simulink library "relay_ANSI_F25_lib"  (Simulink 8.1)
settings: Solver=ode45  StartTime=0.0  StopTime=10.0  RelTol=1e-3
undefined symbols (not defined in the file or in its folder): angle_threshold, dF_threshold, dV_threshold, Ts, VRMSLL
libraries: powerlib_extras x6, simulink_extras x5, simulink x5, dspsigops x2, RMS_lib x1
settings Model: Creator=RE25624  LastModifiedBy=hptb1

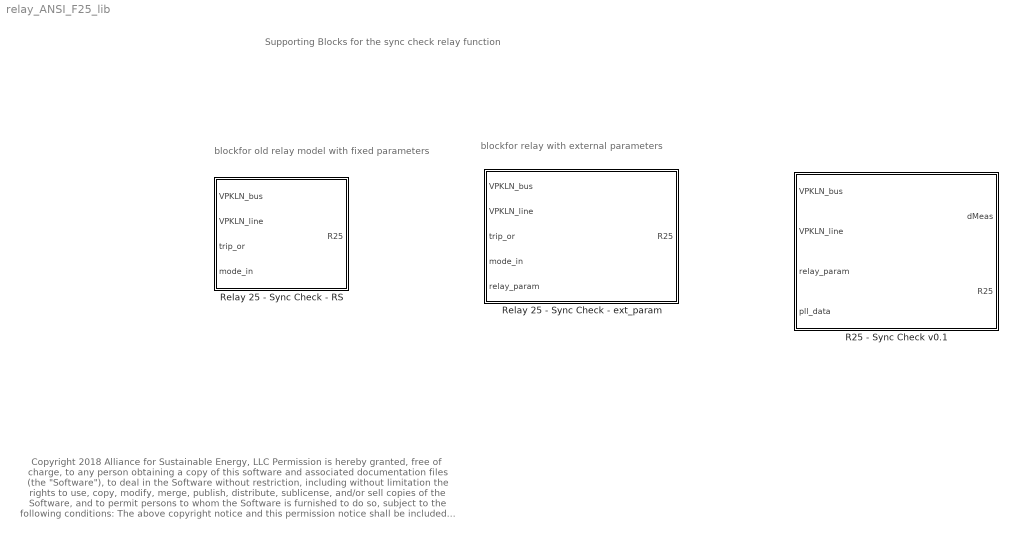
== system relay_ANSI_F25_lib ==
  note: blockfor relay with external parameters
  note: Supporting Blocks for the sync check relay function
  note: blockfor old relay model with fixed parameters
  note: Copyright 2018 Alliance for Sustainable Energy, LLC
      |
      | Permission is hereby granted, free of charge, to any person obtaining a copy of this software
      | and associated documentation files (the "Software"), to deal in the Software without restriction,
      | including without limitation the rights to use, copy, modify, merge, publish, distribute, sublicense,
      | and/or sell copies of the Software, and to permit persons to whom the Software is furnished to do so,
      | subject to the following conditions:
      |
      | The above copyright notice and this permission notice shall be included in all copies or substantial portions of the Software.
      |
      | THE SOFTWARE IS PROVIDED "AS IS", WITHOUT WARRANTY OF ANY KIND, EXPRESS OR IMPLIED, INCLUDING
      | BUT NOT LIMITED TO THE WARRANTIES OF MERCHANTABILITY, FITNESS FOR A PARTICULAR PURPOSE AND
      | NONINFRINGEMENT. IN NO EVENT SHALL THE AUTHORS, THE COPYRIGHT HOLDERS, THE UNITED STATES,
      | THE UNITED STATES DEPARTMENT OF ENERGY, OR ANY OF THEIR EMPLOYEES BE LIABLE FOR ANY CLAIM,
      | DAMAGES OR OTHER LIABILITY, WHETHER IN AN ACTION OF CONTRACT, TORT OR OTHERWISE, ARISING FROM,
      | OUT OF OR IN CONNECTION WITH THE SOFTWARE OR THE USE OR OTHER DEALINGS IN THE SOFTWARE.
  R25 - Sync Check v0.1 : Subsystem  mask(Relay synch check){Ts=Ts}
      mask prompts: Ts "Sampling Time [Sec]"
      mask help:
      | This block checks if the the specified conditions for breaker reclosing
      | are met at both terminals of the circuit breaker. This synch check is
      | intended for use in bus-ties, and service lines.
      |
      | The input bus with the relay parameters should be ordered as follows:
      | 1) VRMSLL
      | 2) IOC
      | 3) TOC
      | 4) dV_threshold
      | 5) angle_threshold
      | 6) dF_threshold
  Relay 25 - Sync Check - RS : Subsystem  mask{VRMSLL=VRMSLL, Ts=Ts, dV_threshold=dV_threshold, angle_threshold=angle_threshold, dF_threshold=dF_threshold}
      mask prompts: VRMSLL "Nominal Voltage [VRMSLL]"; Ts "Sampling Time [Sec]"; dV_threshold "Percent Voltage Threshold [%]"; angle_threshold "Angle Threshold [degress]"; dF_threshold "Frequency Threshold [Hz]"
  Relay 25 - Sync Check - ext_param : Subsystem  mask(Relay synch check){Ts=Ts}
      mask prompts: Ts "Sampling Time [Sec]"
      mask help:
      | This block checks if the the specified conditions for breaker reclosing
      | are met at both terminals of the circuit breaker. This synch check is
      | intended for use in bus-ties, and service lines.
      |
      | The input bus with the relay parameters should be ordered as follows:
      | 1) VRMSLL
      | 2) IOC
      | 3) TOC
      | 4) dV_threshold
      | 5) angle_threshold
      | 6) dF_threshold

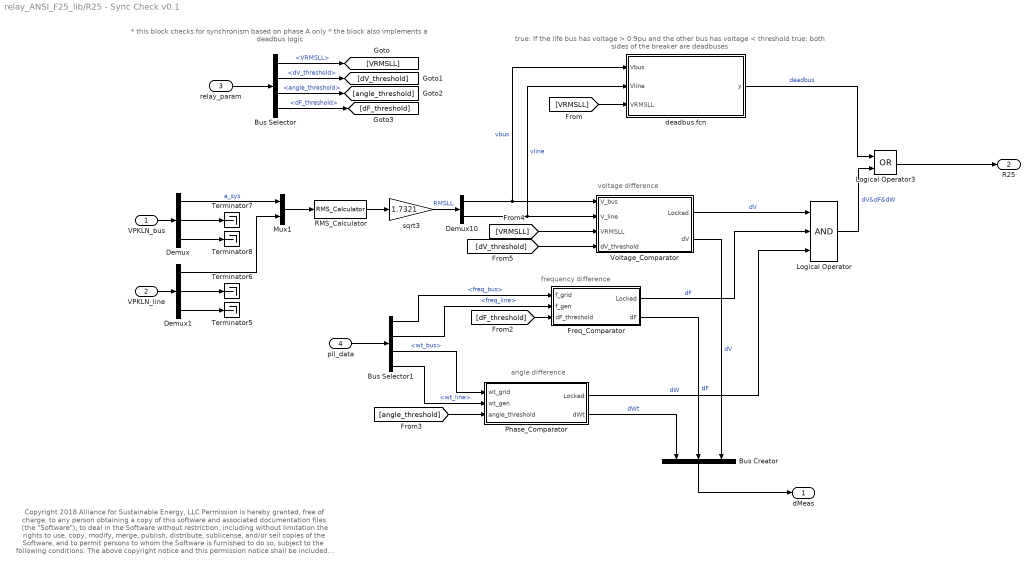
== system relay_ANSI_F25_lib/R25 - Sync Check v0.1 ==
  note: Copyright 2018 Alliance for Sustainable Energy, LLC
      |
      | Permission is hereby granted, free of charge, to any person obtaining a copy of this software
      | and associated documentation files (the "Software"), to deal in the Software without restriction,
      | including without limitation the rights to use, copy, modify, merge, publish, distribute, sublicense,
      | and/or sell copies of the Software, and to permit persons to whom the Software is furnished to do so,
      | subject to the following conditions:
      |
      | The above copyright notice and this permission notice shall be included in all copies or substantial portions of the Software.
      |
      | THE SOFTWARE IS PROVIDED "AS IS", WITHOUT WARRANTY OF ANY KIND, EXPRESS OR IMPLIED, INCLUDING
      | BUT NOT LIMITED TO THE WARRANTIES OF MERCHANTABILITY, FITNESS FOR A PARTICULAR PURPOSE AND
      | NONINFRINGEMENT. IN NO EVENT SHALL THE AUTHORS, THE COPYRIGHT HOLDERS, THE UNITED STATES,
      | THE UNITED STATES DEPARTMENT OF ENERGY, OR ANY OF THEIR EMPLOYEES BE LIABLE FOR ANY CLAIM,
      | DAMAGES OR OTHER LIABILITY, WHETHER IN AN ACTION OF CONTRACT, TORT OR OTHERWISE, ARISING FROM,
      | OUT OF OR IN CONNECTION WITH THE SOFTWARE OR THE USE OR OTHER DEALINGS IN THE SOFTWARE.
  note: true: If the life bus has voltage > 0.9pu and the other bus has voltage < threshold
      | true: both sides of the breaker are deadbuses
  note: voltage difference
  note: frequency difference
  note: angle difference
  note: * this block checks for synchronism based on phase A only
      | * the block also implements a deadbus logic
  VPKLN_bus : Inport
  VPKLN_line : Inport  Port=2
  relay_param : Inport  Port=3
  pll_data : Inport  Port=4
  Bus Creator : BusCreator  Inputs=3
  Bus Selector : BusSelector  OutputSignals=VRMSLL,dV_threshold,angle_threshold,dF_threshold
  Bus Selector1 : BusSelector  OutputSignals=freq_bus,freq_line,wt_bus,wt_line
  Demux : Demux  Outputs=3
  Demux1 : Demux  Outputs=3
  Demux10 : Demux  Outputs=2
  Freq_Comparator : Subsystem
  Logical Operator : Logic  Inputs=3  AllPortsSameDT=off  OutDataTypeStr=boolean
  Logical Operator3 : Logic  Operator=OR  AllPortsSameDT=off  OutDataTypeStr=boolean
  Mux1 : Mux  Inputs=2
  Phase_Comparator : Subsystem
  RMS_Calculator : RMS_lib/RMS_Calculator  Ts=Ts
  Terminator{5..8} (4 alike) : Terminator
  Voltage_Comparator : Subsystem
  deadbus fcn : MATLAB Function  TreatAsAtomicUnit=on
  sqrt3 : Gain  Gain=1.7321
  dMeas : Outport
  R25 : Outport  Port=2
  wires:
  Logical Operator3/1 -> R25/1
  pll_data/1 -> Bus Selector1/1
  Logical Operator/1 -> Logical Operator3/2  "dV&dF&dW"
  deadbus fcn/1(y) -> Logical Operator3/1  "deadbus"
  VPKLN_line/1 -> Demux1/1
  VPKLN_bus/1 -> Demux/1
  Demux/3 -> Terminator8/1
  Demux/2 -> Terminator7/1
  Demux1/3 -> Terminator5/1
  Demux1/2 -> Terminator6/1
  Demux1/1 -> Mux1/2
  Demux/1 -> Mux1/1  "a_sys"
  Demux10/1 -> Voltage_Comparator/1(V_bus), deadbus fcn/1(Vbus)  "vbus"
  Bus Selector1/1 -> Freq_Comparator/1(f_grid)  "<freq_bus>"
  Bus Selector1/2 -> Freq_Comparator/2(f_gen)  "<freq_line>"
  Bus Selector1/3 -> Phase_Comparator/1(wt_grid)  "<wt_bus>"
  Bus Selector1/4 -> Phase_Comparator/2(wt_gen)  "<wt_line>"
  Demux10/2 -> Voltage_Comparator/2(V_line), deadbus fcn/2(Vline)  "vline"
  Voltage_Comparator/1(Locked) -> Logical Operator/1  "dV"
  Freq_Comparator/1(Locked) -> Logical Operator/2  "dF"
  Phase_Comparator/1(Locked) -> Logical Operator/3  "dW"
  RMS_Calculator/1 -> sqrt3/1
  Mux1/1 -> RMS_Calculator/1
  sqrt3/1 -> Demux10/1  "RMSLL"
  [VRMSLL] -> deadbus fcn/3(VRMSLL)
  relay_param/1 -> Bus Selector/1
  Bus Selector/1 -> [VRMSLL]  "<VRMSLL>"
  Bus Selector/2 -> [dV_threshold]  "<dV_threshold>"
  Bus Selector/3 -> [angle_threshold]  "<angle_threshold>"
  Bus Selector/4 -> [dF_threshold]  "<dF_threshold>"
  [dF_threshold] -> Freq_Comparator/3(dF_threshold)
  [angle_threshold] -> Phase_Comparator/3(angle_threshold)
  [VRMSLL] -> Voltage_Comparator/3(VRMSLL)
  [dV_threshold] -> Voltage_Comparator/4(dV_threshold)
  Voltage_Comparator/2(dV) -> Bus Creator/3  "dV"
  Freq_Comparator/2(dF) -> Bus Creator/2  "dF"
  Phase_Comparator/2(dWt) -> Bus Creator/1  "dWt"
  Bus Creator/1 -> dMeas/1

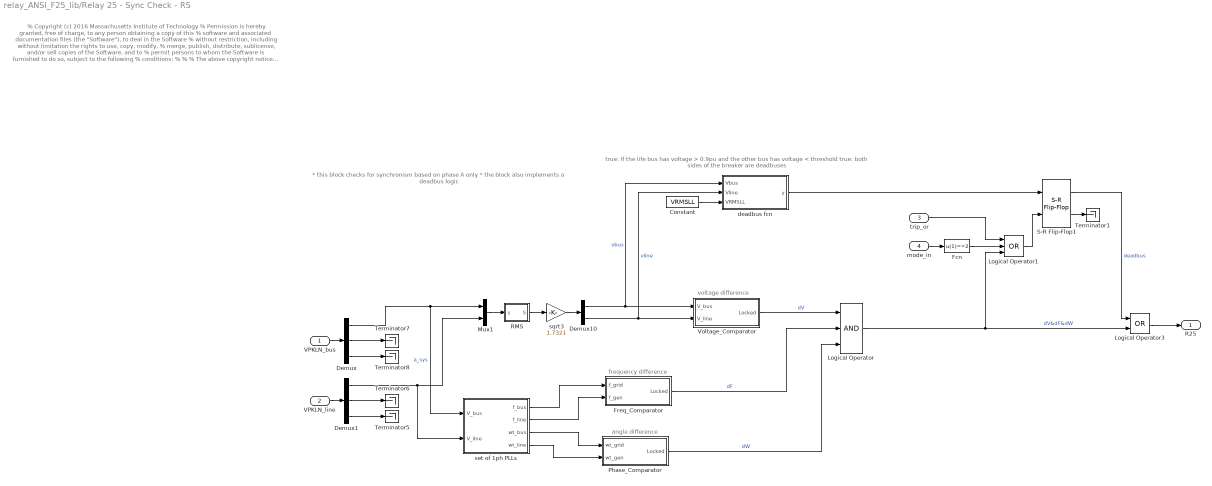
== system relay_ANSI_F25_lib/Relay 25 - Sync Check - RS ==
  note: * this block checks for synchronism based on phase A only
      | * the block also implements a deadbus logic
  note: angle difference
  note: frequency difference
  note: voltage difference
  note: true: If the life bus has voltage > 0.9pu and the other bus has voltage < threshold
      | true: both sides of the breaker are deadbuses
  note: % Copyright (c) 2016 Massachusetts Institute of Technology
      | % Permission is hereby granted, free of charge, to any person obtaining a copy of this
      | % software and associated documentation files (the "Software"), to deal in the Software
      | % without restriction, including without limitation the rights to use, copy, modify,
      | % merge, publish, distribute, sublicense, and/or sell copies of the Software, and to
      | % permit persons to whom the Software is furnished to do so, subject to the following
      | % conditions:
      | %
      | %
      | % The above copyright notice and this permission notice shall be included in
      | % all copies or substantial portions of the Software.
      | %
      | % THE SOFTWARE IS PROVIDED "AS IS", WITHOUT WARRANTY OF ANY KIND, EXPRESS OR IMPLIED,
      | % INCLUDING BUT NOT LIMITED TO THE WARRANTIES OF MERCHANTABILITY, FITNESS FOR A
      | % PARTICULAR PURPOSE AND NONINFRINGEMENT. IN NO EVENT SHALL THE AUTHORS OR COPYRIGHT
      | % HOLDERS BE LIABLE FOR ANY CLAIM, DAMAGES OR OTHER LIABILITY, WHETHER IN AN ACTION
      | % OF CONTRACT, TORT OR OTHERWISE, ARISING FROM, OUT OF OR IN CONNECTION WITH THE
      | % SOFTWARE OR THE USE OR OTHER DEALINGS IN THE SOFTWARE.
      | %
      | %
      | %%
  VPKLN_bus : Inport
  VPKLN_line : Inport  Port=2
  trip_or : Inport  Port=3
  mode_in : Inport  Port=4
  Constant : Constant  Value=VRMSLL
  Demux : Demux  Outputs=3
  Demux1 : Demux  Outputs=3
  Demux10 : Demux  Outputs=2
  Fcn : Fcn  Expr=u(1)==2
  Freq_Comparator : Subsystem
  Logical Operator : Logic  Inputs=3  AllPortsSameDT=off  OutDataTypeStr=boolean
  Logical Operator1 : Logic  Operator=OR  Inputs=3  AllPortsSameDT=off  OutDataTypeStr=boolean
  Logical Operator3 : Logic  Operator=OR  AllPortsSameDT=off  OutDataTypeStr=boolean
  Mux1 : Mux  Inputs=2
  Phase_Comparator : Subsystem
  RMS : Subsystem
  S-R Flip-Flop1 : simulink_extras/Flip Flops/S-R Flip-Flop  initial_condition=0
  Terminator{1,5..8} (5 alike) : Terminator
  Voltage_Comparator : Subsystem
  deadbus fcn : MATLAB Function  TreatAsAtomicUnit=on
  set of 1ph PLLs : Subsystem
  sqrt3 : Gain  Gain=1.7321
  R25 : Outport
  wires:
  Fcn/1 -> Logical Operator1/2
  mode_in/1 -> Fcn/1
  trip_or/1 -> Logical Operator1/1
  Logical Operator1/1 -> S-R Flip-Flop1/2
  deadbus fcn/1(y) -> S-R Flip-Flop1/1
  S-R Flip-Flop1/1 -> Logical Operator3/1  "deadbus"
  Logical Operator3/1 -> R25/1
  S-R Flip-Flop1/2 -> Terminator1/1
  Constant/1 -> deadbus fcn/3(VRMSLL)
  sqrt3/1 -> Demux10/1
  Mux1/1 -> RMS/1(s)
  RMS/1(S) -> sqrt3/1
  Phase_Comparator/1(Locked) -> Logical Operator/3  "dW"
  Freq_Comparator/1(Locked) -> Logical Operator/2  "dF"
  Voltage_Comparator/1(Locked) -> Logical Operator/1  "dV"
  Demux10/2 -> deadbus fcn/2(Vline), Voltage_Comparator/2(V_line)  "vline"
  set of 1ph PLLs/4(wt_line) -> Phase_Comparator/2(wt_gen)
  set of 1ph PLLs/3(wt_bus) -> Phase_Comparator/1(wt_grid)
  set of 1ph PLLs/2(f_line) -> Freq_Comparator/2(f_gen)
  set of 1ph PLLs/1(f_bus) -> Freq_Comparator/1(f_grid)
  Demux10/1 -> deadbus fcn/1(Vbus), Voltage_Comparator/1(V_bus)  "vbus"
  Demux/1 -> Mux1/1, set of 1ph PLLs/1(V_bus)  "a_sys"
  Demux1/1 -> Mux1/2, set of 1ph PLLs/2(V_line)
  Demux1/2 -> Terminator6/1
  Demux1/3 -> Terminator5/1
  Demux/2 -> Terminator7/1
  Demux/3 -> Terminator8/1
  VPKLN_bus/1 -> Demux/1
  VPKLN_line/1 -> Demux1/1
  Logical Operator/1 -> Logical Operator1/3, Logical Operator3/2  "dV&dF&dW"

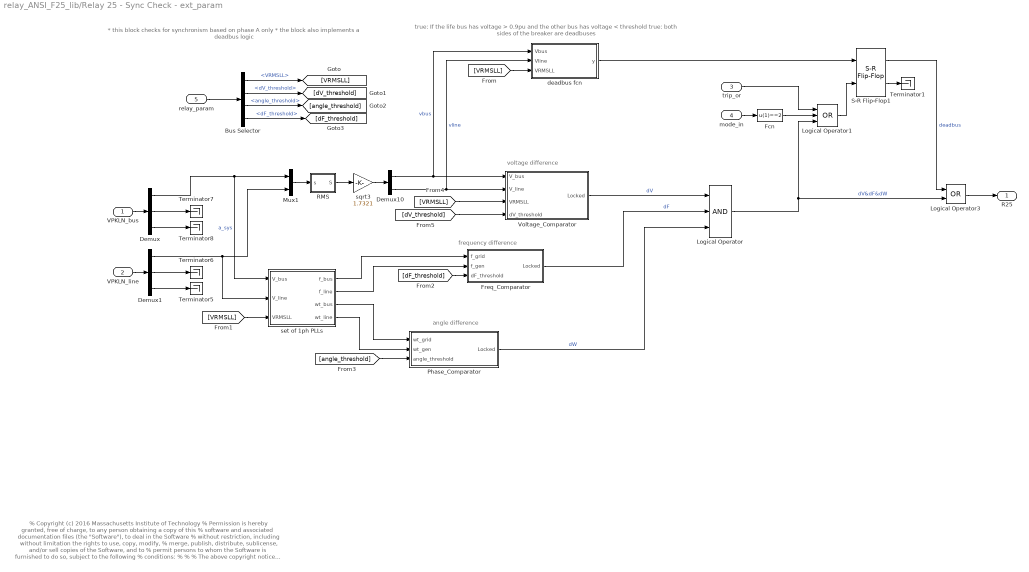
== system relay_ANSI_F25_lib/Relay 25 - Sync Check - ext_param ==
  note: * this block checks for synchronism based on phase A only
      | * the block also implements a deadbus logic
  note: angle difference
  note: frequency difference
  note: voltage difference
  note: true: If the life bus has voltage > 0.9pu and the other bus has voltage < threshold
      | true: both sides of the breaker are deadbuses
  note: % Copyright (c) 2016 Massachusetts Institute of Technology
      | % Permission is hereby granted, free of charge, to any person obtaining a copy of this
      | % software and associated documentation files (the "Software"), to deal in the Software
      | % without restriction, including without limitation the rights to use, copy, modify,
      | % merge, publish, distribute, sublicense, and/or sell copies of the Software, and to
      | % permit persons to whom the Software is furnished to do so, subject to the following
      | % conditions:
      | %
      | %
      | % The above copyright notice and this permission notice shall be included in
      | % all copies or substantial portions of the Software.
      | %
      | % THE SOFTWARE IS PROVIDED "AS IS", WITHOUT WARRANTY OF ANY KIND, EXPRESS OR IMPLIED,
      | % INCLUDING BUT NOT LIMITED TO THE WARRANTIES OF MERCHANTABILITY, FITNESS FOR A
      | % PARTICULAR PURPOSE AND NONINFRINGEMENT. IN NO EVENT SHALL THE AUTHORS OR COPYRIGHT
      | % HOLDERS BE LIABLE FOR ANY CLAIM, DAMAGES OR OTHER LIABILITY, WHETHER IN AN ACTION
      | % OF CONTRACT, TORT OR OTHERWISE, ARISING FROM, OUT OF OR IN CONNECTION WITH THE
      | % SOFTWARE OR THE USE OR OTHER DEALINGS IN THE SOFTWARE.
      | %
      | %
      | %%
  VPKLN_bus : Inport
  VPKLN_line : Inport  Port=2
  trip_or : Inport  Port=3
  mode_in : Inport  Port=4
  relay_param : Inport  Port=5
  Bus Selector : BusSelector  OutputSignals=VRMSLL,dV_threshold,angle_threshold,dF_threshold
  Demux : Demux  Outputs=3
  Demux1 : Demux  Outputs=3
  Demux10 : Demux  Outputs=2
  Fcn : Fcn  Expr=u(1)==2
  Freq_Comparator : Subsystem
  Logical Operator : Logic  Inputs=3  AllPortsSameDT=off  OutDataTypeStr=boolean
  Logical Operator1 : Logic  Operator=OR  Inputs=3  AllPortsSameDT=off  OutDataTypeStr=boolean
  Logical Operator3 : Logic  Operator=OR  AllPortsSameDT=off  OutDataTypeStr=boolean
  Mux1 : Mux  Inputs=2
  Phase_Comparator : Subsystem
  RMS : Subsystem
  S-R Flip-Flop1 : simulink_extras/Flip Flops/S-R Flip-Flop  initial_condition=0
  Terminator{1,5..8} (5 alike) : Terminator
  Voltage_Comparator : Subsystem
  deadbus fcn : MATLAB Function  TreatAsAtomicUnit=on
  set of 1ph PLLs : Subsystem
  sqrt3 : Gain  Gain=1.7321
  R25 : Outport
  wires:
  [dV_threshold] -> Voltage_Comparator/4(dV_threshold)
  [VRMSLL] -> Voltage_Comparator/3(VRMSLL)
  [angle_threshold] -> Phase_Comparator/3(angle_threshold)
  [dF_threshold] -> Freq_Comparator/3(dF_threshold)
  [VRMSLL] -> set of 1ph PLLs/3(VRMSLL)
  Bus Selector/4 -> [dF_threshold]  "<dF_threshold>"
  Bus Selector/3 -> [angle_threshold]  "<angle_threshold>"
  Bus Selector/2 -> [dV_threshold]  "<dV_threshold>"
  Bus Selector/1 -> [VRMSLL]  "<VRMSLL>"
  relay_param/1 -> Bus Selector/1
  Fcn/1 -> Logical Operator1/2
  mode_in/1 -> Fcn/1
  trip_or/1 -> Logical Operator1/1
  Logical Operator1/1 -> S-R Flip-Flop1/2
  deadbus fcn/1(y) -> S-R Flip-Flop1/1
  S-R Flip-Flop1/1 -> Logical Operator3/1  "deadbus"
  Logical Operator3/1 -> R25/1
  S-R Flip-Flop1/2 -> Terminator1/1
  [VRMSLL] -> deadbus fcn/3(VRMSLL)
  sqrt3/1 -> Demux10/1
  Mux1/1 -> RMS/1(s)
  RMS/1(S) -> sqrt3/1
  Phase_Comparator/1(Locked) -> Logical Operator/3  "dW"
  Freq_Comparator/1(Locked) -> Logical Operator/2  "dF"
  Voltage_Comparator/1(Locked) -> Logical Operator/1  "dV"
  Demux10/2 -> deadbus fcn/2(Vline), Voltage_Comparator/2(V_line)  "vline"
  set of 1ph PLLs/4(wt_line) -> Phase_Comparator/2(wt_gen)
  set of 1ph PLLs/3(wt_bus) -> Phase_Comparator/1(wt_grid)
  set of 1ph PLLs/2(f_line) -> Freq_Comparator/2(f_gen)
  set of 1ph PLLs/1(f_bus) -> Freq_Comparator/1(f_grid)
  Demux10/1 -> deadbus fcn/1(Vbus), Voltage_Comparator/1(V_bus)  "vbus"
  Demux/1 -> Mux1/1, set of 1ph PLLs/1(V_bus)  "a_sys"
  Demux1/1 -> Mux1/2, set of 1ph PLLs/2(V_line)
  Demux1/2 -> Terminator6/1
  Demux1/3 -> Terminator5/1
  Demux/2 -> Terminator7/1
  Demux/3 -> Terminator8/1
  VPKLN_bus/1 -> Demux/1
  VPKLN_line/1 -> Demux1/1
  Logical Operator/1 -> Logical Operator1/3, Logical Operator3/2  "dV&dF&dW"

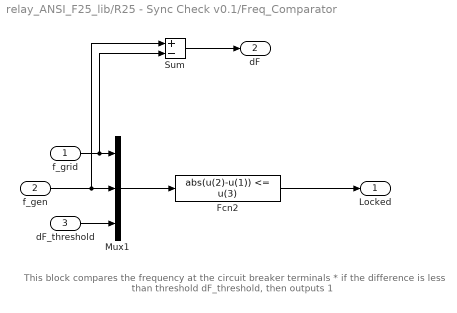
== system relay_ANSI_F25_lib/R25 - Sync Check v0.1/Freq_Comparator ==
  note: This block compares the frequency at the circuit breaker terminals
      | * if the difference is less than threshold dF_threshold, then outputs 1
  f_grid : Inport
  f_gen : Inport  Port=2
  dF_threshold : Inport  Port=3
  Fcn2 : Fcn  Expr=abs(u(2)-u(1)) <= u(3)
  Mux1 : Mux  Inputs=3
  Sum : Sum  Inputs=+-
  Locked : Outport
  dF : Outport  Port=2
  wires:
  Mux1/1 -> Fcn2/1
  Fcn2/1 -> Locked/1
  dF_threshold/1 -> Mux1/3
  f_gen/1 -> Sum/1, Mux1/2
  f_grid/1 -> Sum/2, Mux1/1
  Sum/1 -> dF/1

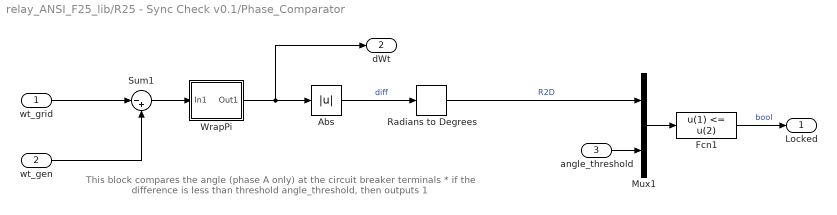
== system relay_ANSI_F25_lib/R25 - Sync Check v0.1/Phase_Comparator ==
  note: This block compares the angle (phase A only) at the circuit breaker terminals
      | * if the difference is less than threshold angle_threshold, then outputs 1
  wt_grid : Inport
  wt_gen : Inport  Port=2
  angle_threshold : Inport  Port=3
  Abs : Abs
  Fcn1 : Fcn  Expr=u(1) <= u(2)  SampleTime=Ts
  Mux1 : Mux  Inputs=2
  Radians to Degrees : simulink_extras/Transformations/Radians to Degrees
  Sum1 : Sum  Inputs=|-+
  WrapPi : Subsystem
  Locked : Outport
  dWt : Outport  Port=2
  wires:
  Abs/1 -> Radians to Degrees/1  "diff"
  Fcn1/1 -> Locked/1  "bool"
  angle_threshold/1 -> Mux1/2
  Mux1/1 -> Fcn1/1
  Radians to Degrees/1 -> Mux1/1  "R2D"
  wt_gen/1 -> Sum1/2
  wt_grid/1 -> Sum1/1
  Sum1/1 -> WrapPi/1(In1)
  WrapPi/1(Out1) -> dWt/1, Abs/1

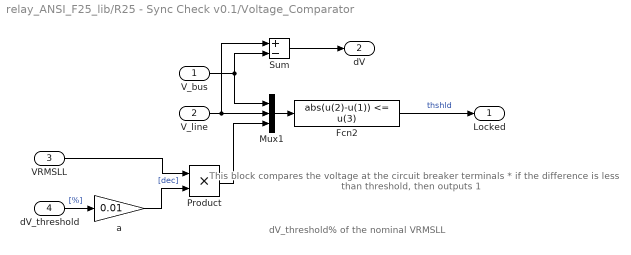
== system relay_ANSI_F25_lib/R25 - Sync Check v0.1/Voltage_Comparator ==
  note: dV_threshold% of the nominal VRMSLL
  note: This block compares the voltage at the circuit breaker terminals
      | * if the difference is less than threshold, then outputs 1
  V_bus : Inport
  V_line : Inport  Port=2
  VRMSLL : Inport  Port=3
  dV_threshold : Inport  Port=4
  Fcn2 : Fcn  Expr=abs(u(2)-u(1)) <= u(3)
  Mux1 : Mux  Inputs=3
  Product : Product
  Sum : Sum  Inputs=+-
  a : Gain  Gain=0.01
  Locked : Outport
  dV : Outport  Port=2
  wires:
  a/1 -> Product/2  "[dec]"
  Mux1/1 -> Fcn2/1
  Fcn2/1 -> Locked/1  "thshld"
  V_line/1 -> Sum/1, Mux1/2
  V_bus/1 -> Mux1/1, Sum/2
  dV_threshold/1 -> a/1  "[%]"
  VRMSLL/1 -> Product/1
  Product/1 -> Mux1/3
  Sum/1 -> dV/1

== system relay_ANSI_F25_lib/Relay 25 - Sync Check - RS/Freq_Comparator ==
  note: This block compares the frequency at each of the circuit breaker terminals
      | * if the difference is less than threshold dF_threshold, then outputs 1
  f_grid : Inport
  f_gen : Inport  Port=2
  Abs : Abs
  Compare To Constant2 : simulink/Logic and Bit Operations/Compare To Constant  relop=<=  const=dF_threshold  OutDataTypeStr=uint8
  Fcn2 : Fcn  Expr=u(2)-u(1)
  Mux1 : Mux  Inputs=2
  Locked : Outport
  wires:
  Compare To Constant2/1 -> Locked/1
  f_grid/1 -> Mux1/1
  f_gen/1 -> Mux1/2
  Fcn2/1 -> Abs/1
  Mux1/1 -> Fcn2/1
  Abs/1 -> Compare To Constant2/1

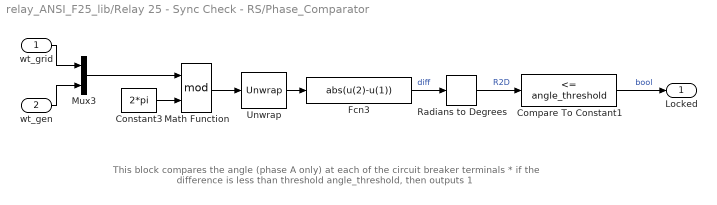
== system relay_ANSI_F25_lib/Relay 25 - Sync Check - RS/Phase_Comparator ==
  note: This block compares the angle (phase A only) at each of the circuit breaker terminals
      | * if the difference is less than threshold angle_threshold, then outputs 1
  wt_grid : Inport
  wt_gen : Inport  Port=2
  Compare To Constant1 : simulink/Logic and Bit Operations/Compare To Constant  relop=<=  const=angle_threshold  OutDataTypeStr=uint8
  Constant3 : Constant  Value=2*pi
  Fcn3 : Fcn  Expr=abs(u(2)-u(1))  SampleTime=Ts
  Math Function : Math  Operator=mod  SampleTime=Ts  SaturateOnIntegerOverflow=on
  Mux3 : Mux  Inputs=2
  Radians to Degrees : simulink_extras/Transformations/Radians to Degrees
  Unwrap : dspsigops/Unwrap  tol=pi  InputProcessing=Columns as channels (frame based)  running=off
  Locked : Outport
  wires:
  Unwrap/1 -> Fcn3/1
  Math Function/1 -> Unwrap/1
  Compare To Constant1/1 -> Locked/1  "bool"
  wt_gen/1 -> Mux3/2
  wt_grid/1 -> Mux3/1
  Fcn3/1 -> Radians to Degrees/1  "diff"
  Mux3/1 -> Math Function/1
  Constant3/1 -> Math Function/2
  Radians to Degrees/1 -> Compare To Constant1/1  "R2D"

== system relay_ANSI_F25_lib/Relay 25 - Sync Check - RS/RMS ==
  s : Inport
  Discrete  Mean value6 : powerlib_extras/Discrete Measurements/Discrete  Mean value  Freq=60  Vinit=0  Ts=Ts
  Product3 : Product  RndMeth=Zero
  Signed Sqrt : Sqrt  SaturateOnIntegerOverflow=on
  S : Outport
  wires:
  Signed Sqrt/1 -> S/1
  Discrete  Mean value6/1 -> Signed Sqrt/1
  Product3/1 -> Discrete  Mean value6/1
  s/1 -> Product3/2, Product3/1

== system relay_ANSI_F25_lib/Relay 25 - Sync Check - RS/Voltage_Comparator ==
  note: This block compares the frequency at each of the circuit breaker terminals
      | * if the difference is less than threshold dF_threshold, then outputs 1
  V_bus : Inport
  V_line : Inport  Port=2
  Fcn2 : Fcn  Expr=abs(u(2)-u(1))
  Mux1 : Mux  Inputs=2
  dV_threshold% of the nominal VRMSLL : simulink/Logic and Bit Operations/Compare To Constant  relop=<=  const=VRMSLL*dV_threshold  OutDataTypeStr=uint8
  Locked : Outport
  wires:
  V_bus/1 -> Mux1/1
  V_line/1 -> Mux1/2
  dV_threshold% of the nominal VRMSLL/1 -> Locked/1  "thshld"
  Fcn2/1 -> dV_threshold% of the nominal VRMSLL/1  "diff"
  Mux1/1 -> Fcn2/1

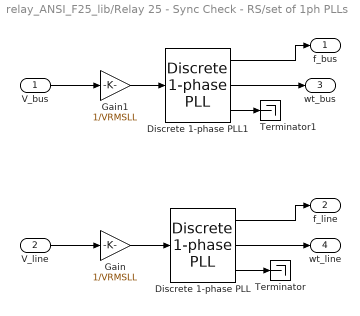
== system relay_ANSI_F25_lib/Relay 25 - Sync Check - RS/set of 1ph PLLs ==
  V_bus : Inport
  V_line : Inport  Port=2
  Discrete 1-phase PLL : powerlib_extras/Discrete  Control Blocks/Discrete 1-phase PLL  Fmin=45  Par_Init=[0 60]  ParK=[ 180 3200 1]  Ts=Ts  AGC=on
  Discrete 1-phase PLL1 : powerlib_extras/Discrete  Control Blocks/Discrete 1-phase PLL  Fmin=45  Par_Init=[0 60]  ParK=[ 180 3200 1]  Ts=Ts  AGC=on
  Gain : Gain  Gain=1/VRMSLL
  Gain1 : Gain  Gain=1/VRMSLL
  Terminator : Terminator
  Terminator1 : Terminator
  f_bus : Outport
  f_line : Outport  Port=2
  wt_bus : Outport  Port=3
  wt_line : Outport  Port=4
  wires:
  Gain1/1 -> Discrete 1-phase PLL1/1
  V_bus/1 -> Gain1/1
  Gain/1 -> Discrete 1-phase PLL/1
  V_line/1 -> Gain/1
  Discrete 1-phase PLL1/1 -> f_bus/1
  Discrete 1-phase PLL1/2 -> wt_bus/1
  Discrete 1-phase PLL/1 -> f_line/1
  Discrete 1-phase PLL/2 -> wt_line/1
  Discrete 1-phase PLL/3 -> Terminator/1
  Discrete 1-phase PLL1/3 -> Terminator1/1

== system relay_ANSI_F25_lib/Relay 25 - Sync Check - ext_param/Freq_Comparator ==
  note: This block compares the frequency at the circuit breaker terminals
      | * if the difference is less than threshold dF_threshold, then outputs 1
  f_grid : Inport
  f_gen : Inport  Port=2
  dF_threshold : Inport  Port=3
  Fcn2 : Fcn  Expr=abs(u(2)-u(1)) <= u(3)
  Mux1 : Mux  Inputs=3
  Locked : Outport
  wires:
  dF_threshold/1 -> Mux1/3
  Fcn2/1 -> Locked/1
  f_grid/1 -> Mux1/1
  f_gen/1 -> Mux1/2
  Mux1/1 -> Fcn2/1

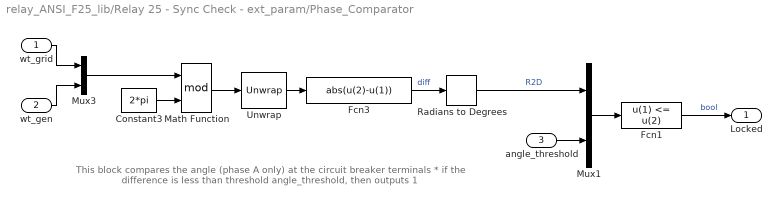
== system relay_ANSI_F25_lib/Relay 25 - Sync Check - ext_param/Phase_Comparator ==
  note: This block compares the angle (phase A only) at the circuit breaker terminals
      | * if the difference is less than threshold angle_threshold, then outputs 1
  wt_grid : Inport
  wt_gen : Inport  Port=2
  angle_threshold : Inport  Port=3
  Constant3 : Constant  Value=2*pi
  Fcn1 : Fcn  Expr=u(1) <= u(2)  SampleTime=Ts
  Fcn3 : Fcn  Expr=abs(u(2)-u(1))  SampleTime=Ts
  Math Function : Math  Operator=mod  SampleTime=Ts  SaturateOnIntegerOverflow=on
  Mux1 : Mux  Inputs=2
  Mux3 : Mux  Inputs=2
  Radians to Degrees : simulink_extras/Transformations/Radians to Degrees
  Unwrap : dspsigops/Unwrap  tol=pi  InputProcessing=Columns as channels (frame based)  running=off
  Locked : Outport
  wires:
  Radians to Degrees/1 -> Mux1/1  "R2D"
  Mux1/1 -> Fcn1/1
  angle_threshold/1 -> Mux1/2
  Unwrap/1 -> Fcn3/1
  Math Function/1 -> Unwrap/1
  Fcn1/1 -> Locked/1  "bool"
  wt_gen/1 -> Mux3/2
  wt_grid/1 -> Mux3/1
  Fcn3/1 -> Radians to Degrees/1  "diff"
  Mux3/1 -> Math Function/1
  Constant3/1 -> Math Function/2

== system relay_ANSI_F25_lib/Relay 25 - Sync Check - ext_param/RMS ==
  s : Inport
  Discrete  Mean value6 : powerlib_extras/Discrete Measurements/Discrete  Mean value  Freq=60  Vinit=0  Ts=Ts
  Product3 : Product  RndMeth=Zero
  Signed Sqrt : Sqrt  SaturateOnIntegerOverflow=on
  S : Outport
  wires:
  Signed Sqrt/1 -> S/1
  Discrete  Mean value6/1 -> Signed Sqrt/1
  Product3/1 -> Discrete  Mean value6/1
  s/1 -> Product3/2, Product3/1

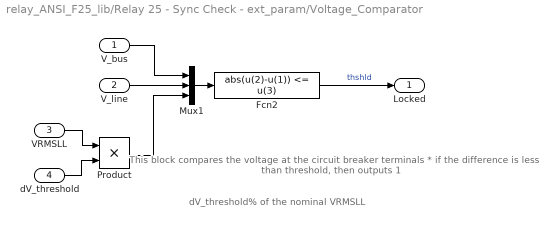
== system relay_ANSI_F25_lib/Relay 25 - Sync Check - ext_param/Voltage_Comparator ==
  note: This block compares the voltage at the circuit breaker terminals
      | * if the difference is less than threshold, then outputs 1
  note: dV_threshold% of the nominal VRMSLL
  V_bus : Inport
  V_line : Inport  Port=2
  VRMSLL : Inport  Port=3
  dV_threshold : Inport  Port=4
  Fcn2 : Fcn  Expr=abs(u(2)-u(1)) <= u(3)
  Mux1 : Mux  Inputs=3
  Product : Product
  Locked : Outport
  wires:
  Product/1 -> Mux1/3
  VRMSLL/1 -> Product/1
  dV_threshold/1 -> Product/2
  V_bus/1 -> Mux1/1
  V_line/1 -> Mux1/2
  Fcn2/1 -> Locked/1  "thshld"
  Mux1/1 -> Fcn2/1

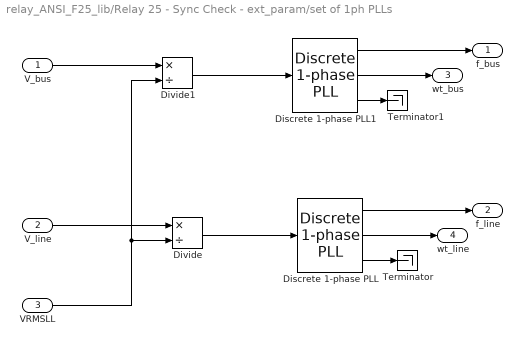
== system relay_ANSI_F25_lib/Relay 25 - Sync Check - ext_param/set of 1ph PLLs ==
  V_bus : Inport
  V_line : Inport  Port=2
  VRMSLL : Inport  Port=3
  Discrete 1-phase PLL : powerlib_extras/Discrete  Control Blocks/Discrete 1-phase PLL  Fmin=45  Par_Init=[0 60]  ParK=[ 180 3200 1]  Ts=Ts  AGC=on
  Discrete 1-phase PLL1 : powerlib_extras/Discrete  Control Blocks/Discrete 1-phase PLL  Fmin=45  Par_Init=[0 60]  ParK=[ 180 3200 1]  Ts=Ts  AGC=on
  Divide : Product  Inputs=*/
  Divide1 : Product  Inputs=*/
  Terminator : Terminator
  Terminator1 : Terminator
  f_bus : Outport
  f_line : Outport  Port=2
  wt_bus : Outport  Port=3
  wt_line : Outport  Port=4
  wires:
  V_bus/1 -> Divide1/1
  Divide1/1 -> Discrete 1-phase PLL1/1
  V_line/1 -> Divide/1
  Divide/1 -> Discrete 1-phase PLL/1
  VRMSLL/1 -> Divide1/2, Divide/2
  Discrete 1-phase PLL1/1 -> f_bus/1
  Discrete 1-phase PLL1/2 -> wt_bus/1
  Discrete 1-phase PLL/1 -> f_line/1
  Discrete 1-phase PLL/2 -> wt_line/1
  Discrete 1-phase PLL/3 -> Terminator/1
  Discrete 1-phase PLL1/3 -> Terminator1/1

== system relay_ANSI_F25_lib/R25 - Sync Check v0.1/Phase_Comparator/WrapPi ==
  In1 : Inport
  Compare To Constant1 : simulink/Logic and Bit Operations/Compare To Constant  relop=<=  const=-pi  OutDataTypeStr=boolean
  Compare To Constant2 : simulink/Logic and Bit Operations/Compare To Constant  relop=>=  const=pi  OutDataTypeStr=boolean
  Gain1 : Gain  Gain=2*pi
  Gain2 : Gain  Gain=2*pi
  Sum : Sum  Inputs=++-
  Out1 : Outport
  wires:
  Sum/1 -> Out1/1
  Gain1/1 -> Sum/1
  Gain2/1 -> Sum/3
  In1/1 -> Compare To Constant2/1, Compare To Constant1/1, Sum/2
  Compare To Constant1/1 -> Gain1/1
  Compare To Constant2/1 -> Gain2/1

== matlab function Relay 25 - Sync Check - ext_param/deadbus fcn ==
  data: Vbus input double; y output double; Vline input double; VRMSLL input double
% Copyright (c) 2016 Massachusetts Institute of Technology
% Permission is hereby granted, free of charge, to any person obtaining a copy of this 
% software and associated documentation files (the "Software"), to deal in the Software
% without restriction, including without limitation the rights to use, copy, modify, 
% merge, publish, distribute, sublicense, and/or sell copies of the Software, and to 
% permit persons to whom the Software is furnished to do so, subject to the following 
% conditions:
% 
% 
% The above copyright notice and this permission notice shall be included in 
% all copies or substantial portions of the Software.
% 
% THE SOFTWARE IS PROVIDED "AS IS", WITHOUT WARRANTY OF ANY KIND, EXPRESS OR IMPLIED, 
% INCLUDING BUT NOT LIMITED TO THE WARRANTIES OF MERCHANTABILITY, FITNESS FOR A 
% PARTICULAR PURPOSE AND NONINFRINGEMENT. IN NO EVENT SHALL THE AUTHORS OR COPYRIGHT 
% HOLDERS BE LIABLE FOR ANY CLAIM, DAMAGES OR OTHER LIABILITY, WHETHER IN AN ACTION 
% OF CONTRACT, TORT OR OTHERWISE, ARISING FROM, OUT OF OR IN CONNECTION WITH THE 
% SOFTWARE OR THE USE OR OTHER DEALINGS IN THE SOFTWARE.
%
%
%%

function y = fcn(Vbus, Vline, VRMSLL)
%#codegen
if isnan(Vbus)
    Vbus=0;
elseif isnan(Vline)
    Vline = 0;
end

% voltage threshold for deadbus
if VRMSLL > 400
    threshold = VRMSLL * 0.003; % @ 0.3%
else
    threshold = VRMSLL * 0.05; % @ 5%
end

% bounding open-circuit voltage at 120%
a = (Vbus>(VRMSLL*0.90)) && (Vbus<(VRMSLL*1.20)) && (Vline < threshold);
b = (Vline>(VRMSLL*0.90)) && (Vline<(VRMSLL*1.20)) && (Vbus < threshold);
c = (Vline < threshold) && (Vbus < threshold);
y = a||b||c;

== matlab function R25 - Sync Check v0.1/deadbus fcn ==
  data: Vbus input double; y output double; Vline input double; VRMSLL input double
% Copyright (c) 2016 Massachusetts Institute of Technology
% Permission is hereby granted, free of charge, to any person obtaining a copy of this
% software and associated documentation files (the "Software"), to deal in the Software
% without restriction, including without limitation the rights to use, copy, modify,
% merge, publish, distribute, sublicense, and/or sell copies of the Software, and to
% permit persons to whom the Software is furnished to do so, subject to the following
% conditions:
%
%
% The above copyright notice and this permission notice shall be included in
% all copies or substantial portions of the Software.
%
% THE SOFTWARE IS PROVIDED "AS IS", WITHOUT WARRANTY OF ANY KIND, EXPRESS OR IMPLIED,
% INCLUDING BUT NOT LIMITED TO THE WARRANTIES OF MERCHANTABILITY, FITNESS FOR A
% PARTICULAR PURPOSE AND NONINFRINGEMENT. IN NO EVENT SHALL THE AUTHORS OR COPYRIGHT
% HOLDERS BE LIABLE FOR ANY CLAIM, DAMAGES OR OTHER LIABILITY, WHETHER IN AN ACTION
% OF CONTRACT, TORT OR OTHERWISE, ARISING FROM, OUT OF OR IN CONNECTION WITH THE
% SOFTWARE OR THE USE OR OTHER DEALINGS IN THE SOFTWARE.
%
%
%%

function y = fcn(Vbus, Vline, VRMSLL)
%#codegen
if isnan(Vbus)
    Vbus=0;
elseif isnan(Vline)
    Vline = 0;
end

% voltage threshold for deadbus
if VRMSLL > 520
    threshold = VRMSLL * 0.03; % @ 3%
else
    threshold = VRMSLL * 0.05; % @ 5%
end

% selecting 10V as the deadbus band - similar to SEL751
% threshold = 10;

% bounding open-circuit voltage at 120%
a = (Vbus>(VRMSLL*0.8)) && (Vbus<(VRMSLL*1.20)) && (Vline < threshold);
b = (Vline>(VRMSLL*0.8)) && (Vline<(VRMSLL*1.20)) && (Vbus < threshold);
c = (Vline < threshold) && (Vbus < threshold);
y = a||b||c;

== matlab function Relay 25 - Sync Check - RS/deadbus fcn ==
  data: Vbus input double; y output double; Vline input double; VRMSLL input double
% Copyright (c) 2016 Massachusetts Institute of Technology
% Permission is hereby granted, free of charge, to any person obtaining a copy of this 
% software and associated documentation files (the "Software"), to deal in the Software
% without restriction, including without limitation the rights to use, copy, modify, 
% merge, publish, distribute, sublicense, and/or sell copies of the Software, and to 
% permit persons to whom the Software is furnished to do so, subject to the following 
% conditions:
% 
% 
% The above copyright notice and this permission notice shall be included in 
% all copies or substantial portions of the Software.
% 
% THE SOFTWARE IS PROVIDED "AS IS", WITHOUT WARRANTY OF ANY KIND, EXPRESS OR IMPLIED, 
% INCLUDING BUT NOT LIMITED TO THE WARRANTIES OF MERCHANTABILITY, FITNESS FOR A 
% PARTICULAR PURPOSE AND NONINFRINGEMENT. IN NO EVENT SHALL THE AUTHORS OR COPYRIGHT 
% HOLDERS BE LIABLE FOR ANY CLAIM, DAMAGES OR OTHER LIABILITY, WHETHER IN AN ACTION 
% OF CONTRACT, TORT OR OTHERWISE, ARISING FROM, OUT OF OR IN CONNECTION WITH THE 
% SOFTWARE OR THE USE OR OTHER DEALINGS IN THE SOFTWARE.
%
%
%%

function y = fcn(Vbus, Vline, VRMSLL)
%#codegen
if isnan(Vbus)
    Vbus=0;
elseif isnan(Vline)
    Vline = 0;
end

% voltage threshold for deadbus
if VRMSLL > 400
    threshold = VRMSLL * 0.003; % @ 0.3%
else
    threshold = VRMSLL * 0.05; % @ 5%
end

% bounding open-circuit voltage at 120%
a = (Vbus>(VRMSLL*0.90)) && (Vbus<(VRMSLL*1.20)) && (Vline < threshold);
b = (Vline>(VRMSLL*0.90)) && (Vline<(VRMSLL*1.20)) && (Vbus < threshold);
c = (Vline < threshold) && (Vbus < threshold);
y = a||b||c;
